simulink model "BMS_project"  (R2022a)
settings: Solver=VariableStepAuto  StartTime=0.0  StopTime=100  RelTol=1e-3
undefined symbols (not defined in the file): Ion, Lithium
libraries: spsIdealSwitchLib x2, spsBatteryLib x1, spsDCVoltageSourceLib x1, spsSeriesRLCLoadLib x1, spspowerguiLib x1
settings Model: Creator=prudh  LastModifiedBy=my pc
settings DebuggingCC: UnconnectedInputMsg=warning  UnconnectedOutputMsg=warning  UnconnectedLineMsg=warning
settings RTWCC: DLArmComputeVersion=19.05

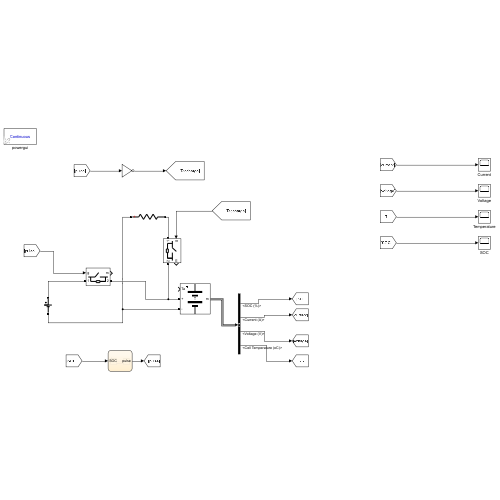
[thumbnail: Simulink's stored preview of the top-level diagram]
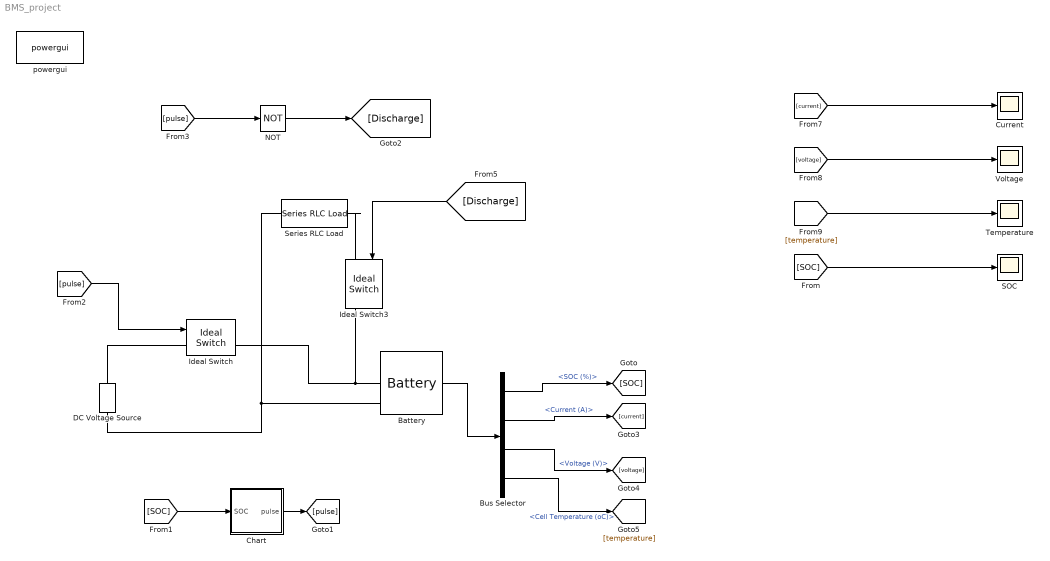
== system BMS_project ==
  Battery : spsBatteryLib/Battery  BatType=Lithium-Ion  ShowTempParam=on  ThermalPreset="3.3V  2.3Ah  (LiFePO4)"  ShowAgeParam=off  NomV=3.3  NomQ=2.3  SOC=10  Batt_Tr=50  PresetModel=off  MaxQ=2.3  MinV=2.475  FullV=3.748  Dis_rate=2.3  R=0.014  Normal_OP=2.25  expZone="[3.4788       0.113]"  current=[6.5 13 32.5]  Units=Time  Tci=20  NomT=25  T2=0  MaxQ2=2.208  FullV2=3.45  Normal_OP2=2.85  expZone2="[3.22       0.015]"  Rca=0.6  ti=1000  Dp=0  Neq0=0  Tsim=1e6  Ta1=25  Qeol=5.4*0.9  Reol=0.013333*1.2  Char_age=[2.3478, 3]  Dis_age=[2.3478, 10]  N1=1500  N2=10500  N3=1000  N4=1400  Ta2=45  N5=950
  Bus Selector : BusSelector  OutputSignals=SOC (%),Current (A),Voltage (V),Cell Temperature (oC)
  Chart : Stateflow chart  TreatAsAtomicUnit=on
  Current : Scope
  DC Voltage Source : spsDCVoltageSourceLib/DC Voltage Source  Amplitude=15  Measurements=None
  Ideal Switch : spsIdealSwitchLib/Ideal Switch  Ron=0.001  Lon=0  IC=0  Rs=1e5  Cs=inf  Measurements=on
  Ideal Switch3 : spsIdealSwitchLib/Ideal Switch  Ron=0.001  Lon=0  IC=0  Rs=1e5  Cs=inf  Measurements=on
  NOT : Logic  Operator=NOT  IconShape=distinctive  AllPortsSameDT=off  OutDataTypeStr=boolean
  SOC : Scope
  Series RLC Load : spsSeriesRLCLoadLib/Series RLC Load  LConnTagsString=a  RConnTagsString=__new0  NominalVoltage=10  NominalFrequency=60  ActivePower=1000  InductivePower=0  CapacitivePower=0  Setx0=off  InitialVoltage=0  SetiL0=off  InitialCurrent=0  Measurements=None  LoadType=constant Z
  Temperature : Scope
  Voltage : Scope
  powergui : spspowerguiLib/powergui  Priority=1  SimulationMode=Continuous  SampleTime=50e-6  frequency=60  Iterations=50  frequencyindice=0  Pbase=100e6  ErrMax=1e-4  UnitsV=kV  UnitsW=MW  buscounter=0  FunctionMessages=off  echomessages=off  EnableUseOfTLC=off  CurrentSourceSwitches=off  DisableSnubberDevices=off  DisableRonSwitches=off  DisableVfSwitches=off  DisplayEquations=off  AutomaticDiscreteSolvers=off  SolverType=Tustin/Backward Euler (TBE)  Interpol=off  ExternalGateDelay=off  methode=off  Ts=100  x0status=blocks  SPID=on  SwTol=0  HookPort=off  NonlinearTolerance=1e-4  nMaxIteration=100  ContinueOnMaxIteration=off  RestoreLinks=warning  ResistiveCurrentMeasurement=off  Frange=[0:2:500]  Ylog=off  Xlog=on  ShowGrid=off  save=off  variable=ZData  structure=0  ZoomFFT=off  StartTime=0.0  cycles=1  DisplayStyle=1  fundamental=60  FreqAxis=off  MaxFrequency=1000  frequencyindicesteady=1  RmsSteady=1  display=off
  wires:
  [current] -> Current/1
  [SOC] -> SOC/1
  [voltage] -> Voltage/1
  Bus Selector/2 -> [current]  "<Current (A)>"
  Bus Selector/3 -> [voltage]  "<Voltage (V)>"
  Bus Selector/1 -> [SOC]  "<SOC (%)>"
  [Discharge] -> Ideal Switch3/1
  [pulse] -> Ideal Switch/1
  Chart/1(pulse) -> [pulse]
  NOT/1 -> [Discharge]
  [SOC] -> Chart/1(SOC)
  Bus Selector/4 -> [temperature]  "<Cell Temperature (oC)>"
  [pulse] -> NOT/1
  [temperature] -> Temperature/1
  Battery/1 -> Bus Selector/1
  connections:
  Series RLC Load/RConn1 -- Ideal Switch3/LConn1
  DC Voltage Source/LConn1 -- Series RLC Load/LConn1 -- Battery/LConn2
  Ideal Switch/LConn1 -- DC Voltage Source/RConn1
  Ideal Switch/RConn1 -- Ideal Switch3/RConn1 -- Battery/LConn1

== stateflow chart BMS_project/Chart ==
  state Charge
    entry:pulse=1
  state discharge
    entry:pulse=0
  (default) -> Charge
  Charge -> discharge : [SOC>80]
  discharge -> Charge : [SOC<40]
  data: SOC input; pulse output
